simulink model "model_MD_gaslift"  (R2023a)
settings: Solver=ode15s  StartTime=0  StopTime=par.simulation_time  FixedStep=par.sample_time  RelTol=1e-3
values from neighbouring files (symbols this model uses):
  par = function_parameters_MPC_MD_gaslift    [main_MPC_MD_gaslift.m]
settings Model: Creator=aslik  LastModifiedBy=aslik
settings DataIOCC: SaveOutput=off  SignalLogging=off  DSMLogging=off  StreamToWks=off  SaveTime=off  ReturnWorkspaceOutputs=off  DatasetSignalFormat=timetable
settings OptimizationCC: BlockReduction=off  OptimizeBlockIOStorage=off  BufferReuse=off
settings DebuggingCC: AlgebraicLoopMsg=none
settings ModelReferenceCC: EnableRefExpFcnMdlSchedulingChecks=on
settings RTWCC: DLArmComputeVersion=19.05

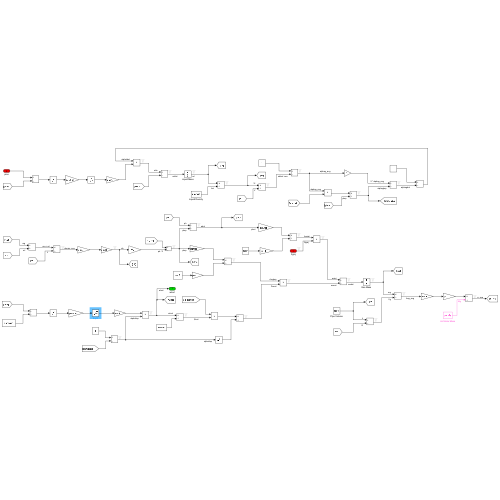
[thumbnail: Simulink's stored preview of the top-level diagram]
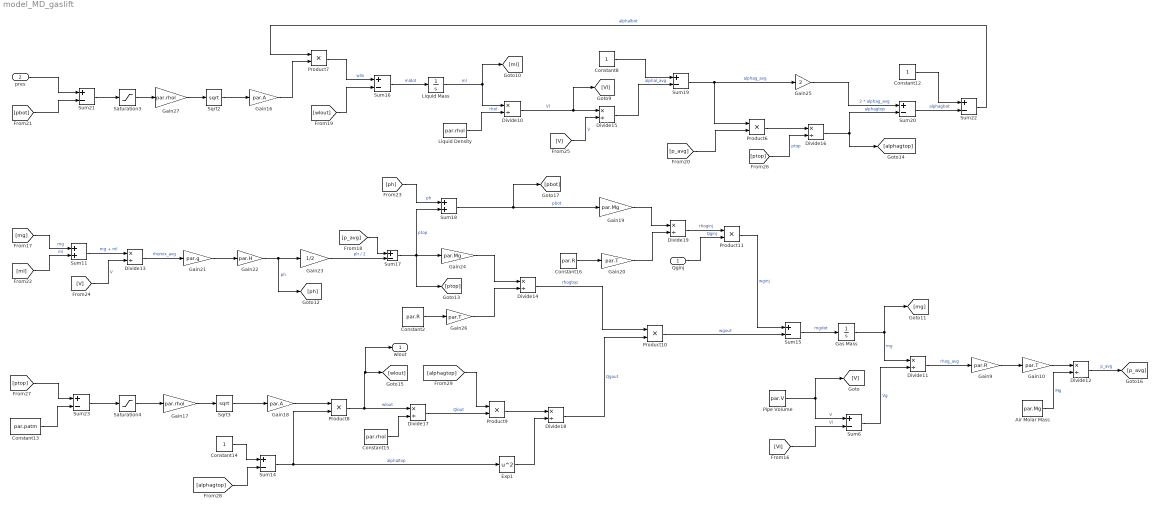
== system model_MD_gaslift ==
  Qginj : Inport
  pres : Inport  Port=2
  Air Molar Mass : Constant  Value=par.Mg  OutDataTypeStr=double
  Constant12 : Constant  OutDataTypeStr=double
  Constant13 : Constant  Value=par.patm  OutDataTypeStr=double
  Constant14 : Constant  OutDataTypeStr=double
  Constant15 : Constant  Value=par.rhol  OutDataTypeStr=double
  Constant16 : Constant  Value=par.R  OutDataTypeStr=double
  Constant2 : Constant  Value=par.R  OutDataTypeStr=double
  Constant8 : Constant  OutDataTypeStr=double
  Divide{10..19} (10 alike) : Product  Inputs=*/
  Exp1 : Math  Operator=square
  Gain10 : Gain  Gain=par.T
  Gain16 : Gain  Gain=par.A
  Gain17 : Gain  Gain=par.rhol
  Gain18 : Gain  Gain=par.A
  Gain19 : Gain  Gain=par.Mg
  Gain20 : Gain  Gain=par.T
  Gain21 : Gain  Gain=par.g
  Gain22 : Gain  Gain=par.H
  Gain23 : Gain  Gain=1/2
  Gain24 : Gain  Gain=par.Mg
  Gain25 : Gain  Gain=2
  Gain26 : Gain  Gain=par.T
  Gain27 : Gain  Gain=par.rhol
  Gain9 : Gain  Gain=par.R
  "Gas Mass " : Integrator  InitialCondition=par.mg0  LowerSaturationLimit=0  ContinuousStateAttributes='mg'
  Liquid Density : Constant  Value=par.rhol  OutDataTypeStr=double
  Liquid Mass : Integrator  InitialCondition=par.ml0  LowerSaturationLimit=0  ContinuousStateAttributes='ml'
  Pipe Volume : Constant  Value=par.V  OutDataTypeStr=double
  Product{6..11} (6 alike) : Product
  Saturation3 : Saturate  UpperLimit=inf  LowerLimit=0
  Saturation4 : Saturate  UpperLimit=inf  LowerLimit=0
  Sqrt2 : Sqrt  OutDataTypeStr=double  IntermediateResultsDataTypeStr=double
  Sqrt3 : Sqrt  OutDataTypeStr=double  IntermediateResultsDataTypeStr=double
  Sum11 : Sum
  Sum{6,14..17,19..23} (10 alike) : Sum  Inputs=+-
  Sum18 : Sum
  wlout : Outport
  wires:
  Product6/1 -> Divide16/1
  Divide10/1 -> Divide15/1, [Vl]  "Vl"
  Constant12/1 -> Sum22/1
  Gain24/1 -> Divide14/1
  Sum11/1 -> Divide13/1  "mg + ml"
  Divide14/1 -> Product10/1  "rhogtop"
  Gain9/1 -> Gain10/1
  pres/1 -> Sum21/1
  Constant13/1 -> Sum23/2
  [Vl] -> Sum6/2  "Vl"
  Qginj/1 -> Product11/2  "Qginj"
  Saturation3/1 -> Gain27/1
  Sum15/1 -> "Gas Mass "/1  "mgdot"
  Sum18/1 -> [pbot], Gain19/1  "pbot"
  [alphagtop] -> Product9/1
  Divide18/1 -> Product10/2  "Qgout"
  Exp1/1 -> Divide18/2
  Gain27/1 -> Sqrt2/1
  Gain23/1 -> Sum17/2  "ph / 2"
  Gain16/1 -> Product7/2
  Product7/1 -> Sum16/1  "wlin"
  Gain21/1 -> Gain22/1
  Sqrt3/1 -> Gain18/1
  Gain17/1 -> Sqrt3/1
  Divide16/1 -> [alphagtop], Sum20/2  "alphagtop"
  Gain18/1 -> Product8/1
  Divide13/1 -> Gain21/1  "rhomix_avg"
  Sum19/1 -> Product6/1, Gain25/1  "alphag_avg"
  Constant8/1 -> Sum19/1
  [p_avg] -> Sum17/1
  Sum22/1 -> Product7/1  "alphalbot"
  Product11/1 -> Sum15/1  "wginj"
  Constant14/1 -> Sum14/1
  [ptop] -> Divide16/2  "ptop"
  Constant2/1 -> Gain26/1
  Gain26/1 -> Divide14/2
  Air Molar Mass/1 -> Divide12/2  "Mg"
  Gain25/1 -> Sum20/1  "2 * alphag_avg"
  Liquid Density/1 -> Divide10/2  "rhol"
  [pbot] -> Sum21/2
  Product9/1 -> Divide18/1
  Sum23/1 -> Saturation4/1
  Gain10/1 -> Divide12/1
  Divide12/1 -> [p_avg]  "p_avg"
  Gain20/1 -> Divide19/2
  Sum20/1 -> Sum22/2  "alphagbot"
  Gain22/1 -> [ph], Gain23/1  "ph"
  Divide17/1 -> Product9/2  "Qlout"
  [alphagtop] -> Sum14/2
  [ph] -> Sum18/1  "ph"
  Constant16/1 -> Gain20/1
  Divide11/1 -> Gain9/1  "rhog_avg"
  Constant15/1 -> Divide17/2
  [ml] -> Sum11/2  "ml"
  Sum14/1 -> Product8/2, Exp1/1  "alphaltop"
  Saturation4/1 -> Gain17/1
  Sqrt2/1 -> Gain16/1
  Liquid Mass/1 -> [ml], Divide10/1  "ml"
  Divide19/1 -> Product11/1  "rhoginj"
  Sum16/1 -> Liquid Mass/1  "mldot"
  Pipe Volume/1 -> [V], Sum6/1  "V"
  [V] -> Divide15/2  "V"
  [mg] -> Sum11/1  "mg"
  "Gas Mass "/1 -> [mg], Divide11/1  "mg"
  [ptop] -> Sum23/1
  [wlout] -> Sum16/2
  Sum6/1 -> Divide11/2  "Vg"
  Sum17/1 -> Gain24/1, Sum18/2, [ptop]  "ptop"
  Product8/1 -> wlout/1, [wlout], Divide17/1  "wlout"
  Sum21/1 -> Saturation3/1
  [p_avg] -> Product6/2
  Product10/1 -> Sum15/2  "wgout"
  Gain19/1 -> Divide19/1
  [V] -> Divide13/2  "V"
  Divide15/1 -> Sum19/2  "alphal_avg"
